simulink model "symblock"  (Simulink 9.1)
settings: Solver=ode45  StartTime=0.0  StopTime=Tsim  FixedStep=T  RelTol=1e-3  EnableMultiTasking=on
values from neighbouring files (symbols this model uses):
  b = 20    [hd.m]
  D = 0    [hd.m]
  J = 1    [hd.m]
  Km = 5    [hd.m]
  L = 10^-3    (= 0.001)    [hd.m]
  R = 1    [hd.m]
  T = 0.1    [hd.m]
  W = 1    [hd.m]
settings Model: Creator=hcf2k  LastModifiedBy=Rodrigo
settings DataIOCC: LimitDataPoints=on  SaveFormat=StructureWithTime  SignalLoggingSaveFormat=ModelDataLogs
settings DebuggingCC: UnderspecifiedInitializationDetection=Simplified  MergeDetectMultiDrivingBlocksExec=error  FcnCallInpInsideContextMsg=warning
settings HardwareCC: ProdIntDivRoundTo=Zero  ProdEndianess=LittleEndian  ProdHWDeviceType=Specified

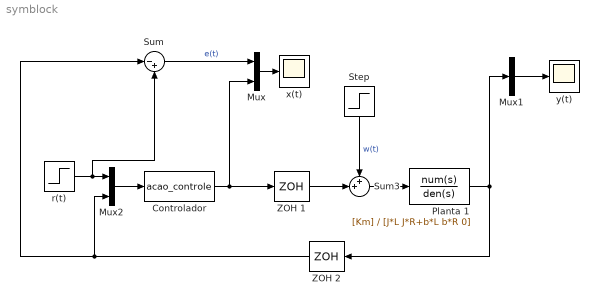
== system symblock ==
  Controlador : MATLABFcn  MATLABFcn=acao_controle  OutputDimensions=1
  Mux : Mux  Inputs=2
  Mux1 : Mux  Inputs=1
  Mux2 : Mux  Inputs=2
  Planta 1 : TransferFcn  Numerator=[Km]  Denominator=[J*L J*R+b*L b*R 0]
  Step : Step  Time=0  After=W  SampleTime=0
  Sum : Sum  Inputs=|-+
  Sum3 : Sum  Inputs=++|
  ZOH 1 : ZeroOrderHold  SampleTime=T
  ZOH 2 : ZeroOrderHold  SampleTime=T
  r(t) : Step  Time=0  After=D  SampleTime=T
  x(t) : Scope
  y(t) : Scope
  wires:
  Mux1/1 -> y(t)/1
  Planta 1/1 -> Mux1/1, ZOH 2/1
  Controlador/1 -> Mux/2, ZOH 1/1
  Mux/1 -> x(t)/1
  r(t)/1 -> Sum/2, Mux2/1
  Mux2/1 -> Controlador/1
  ZOH 2/1 -> Mux2/2, Sum/1
  Sum/1 -> Mux/1  "e(t)"
  Sum3/1 -> Planta 1/1
  Step/1 -> Sum3/1  "w(t)"
  ZOH 1/1 -> Sum3/2
